simulink model "modal_control_with_integrator_open_loop_system"  (R2020b)
settings: Solver=VariableStepAuto  StartTime=0.0  StopTime=200  RelTol=1e-3
values from neighbouring files (symbols this model uses):
  COUPLING_COEFFICIENT = 0.5736    [Workshop_MATLAB.m]
  ESTIMATOR_TRANSFER_FUNCTION_DENOMINATOR = [ESTIMATOR_TIME_CONSTANT 1]    [Workshop_MATLAB.m]
  ESTIMATOR_TRANSFER_FUNCTION_NUMERATOR = [1 0]    [Workshop_MATLAB.m]
  FLEXIBLE_MODE_DAMPING_RATIO = 0.00495    [Workshop_MATLAB.m]
  FLEXIBLE_MODE_FREQUENCY = 2.6268    [Workshop_MATLAB.m]
  INITIAL_CONDITION_ON_STATE = 0.0001    [Workshop_MATLAB.m]
  SATELLITE_INERTIA = 31.38    [Workshop_MATLAB.m]
  SMALL_POINTING_ERROR = 0.5*2*pi/360    (= 0.00872664625997)    [Workshop_MATLAB.m]
undefined symbols (not defined in the file or in its folder): REACTION_WHEEL_REDUCED_FORM
settings Model: Creator=WLCG  LastModifiedBy=WLCG

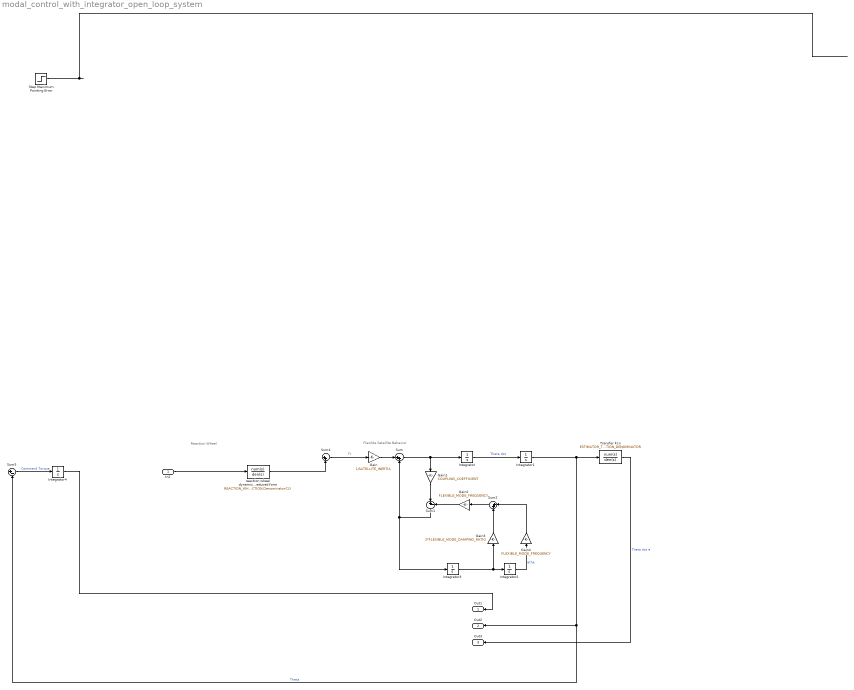
== system modal_control_with_integrator_open_loop_system ==
  note: Reaction Wheel
  note: Flexible Satellite Behavior
  In2 : Inport
  Gain : Gain  Gain=1/SATELLITE_INERTIA
  Gain1 : Gain  Gain=COUPLING_COEFFICIENT
  Gain2 : Gain  Gain=FLEXIBLE_MODE_FREQUENCY
  Gain3 : Gain  Gain=2*FLEXIBLE_MODE_DAMPING_RATIO
  Gain4 : Gain  Gain=FLEXIBLE_MODE_FREQUENCY
  Integrator{,1,3..4} (4 alike) : Integrator
  Integrator2 : Integrator  InitialCondition=INITIAL_CONDITION_ON_STATE
  Step Maximum Pointing Error : Step  Time=0  After=SMALL_POINTING_ERROR  SampleTime=0
  Sum : Sum  Inputs=|++
  Sum1 : Sum  Inputs=|+-
  Sum2 : Sum  Inputs=|++
  Sum4 : Sum  Inputs=|++
  Sum5 : Sum  Inputs=|+-
  Transfer Fcn : TransferFcn  Numerator=ESTIMATOR_TRANSFER_FUNCTION_NUMERATOR  Denominator=ESTIMATOR_TRANSFER_FUNCTION_DENOMINATOR
  reaction wheel dynamics reduced form : TransferFcn  Numerator=REACTION_WHEEL_REDUCED_FORM.TRANSFER_FUNCTION.Numerator{1}  Denominator=REACTION_WHEEL_REDUCED_FORM.TRANSFER_FUNCTION.Denominator{1}
  Out1 : Outport
  Out2 : Outport  Port=2
  Out3 : Outport  Port=3
  wires:
  Sum2/1 -> Gain2/1
  Gain4/1 -> Sum2/1
  Integrator3/1 -> Integrator2/1, Gain3/1
  Integrator1/1 -> Sum5/2, Out2/1, Transfer Fcn/1  "Theta"
  Gain1/1 -> Sum1/1
  Sum4/1 -> Gain/1  "Tr"
  Integrator2/1 -> Gain4/1  "etha"
  reaction wheel dynamics reduced form/1 -> Sum4/2
  Gain2/1 -> Sum1/2
  Sum/1 -> Gain1/1, Integrator/1
  Integrator/1 -> Integrator1/1  "Theta dot"
  Gain3/1 -> Sum2/2
  Sum1/1 -> Sum/2, Integrator3/1
  Gain/1 -> Sum/1
  Sum5/1 -> Integrator4/1  "Command Torque"
  Integrator4/1 -> Out1/1
  Transfer Fcn/1 -> Out3/1  "Theta dot e"
  In2/1 -> reaction wheel dynamics reduced form/1
  Step Maximum Pointing Error/1 -> ?
